simulink library "dlbsBlockSqrt"  (R2025b)
settings: Solver=VariableStepAuto  StartTime=0.0  StopTime=10.0  RelTol=1e-3
libraries: dlbsBlockExtractGradientGF x1, dlbsBlockInsertGradientGF x1
settings Model: Creator=lt6037  LastModifiedBy=lt6037

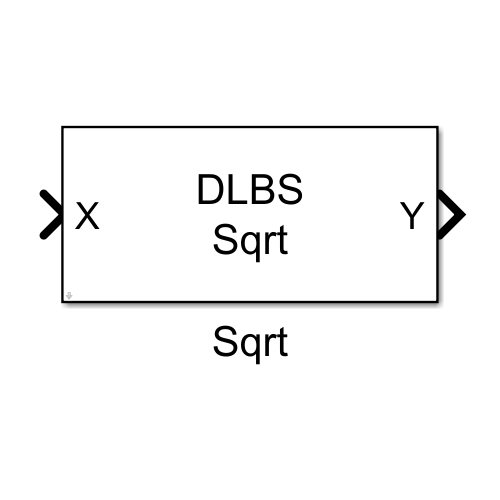
[thumbnail: Simulink's stored preview of the top-level diagram]
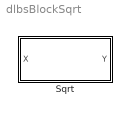
== system dlbsBlockSqrt ==
  Sqrt : Subsystem
      mask help: Applies the square root to the input tensor. The operation is applied element-wise across all tensor elements.
      mask Help: web("dlbsHelpBlockSqrt.html")
      mask Display: fprintf("DLBS\nSqrt");

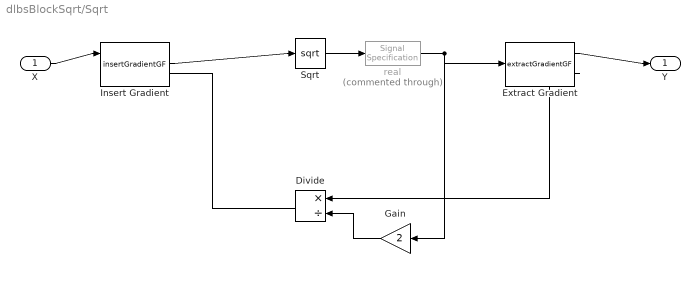
== system dlbsBlockSqrt/Sqrt ==
  X : Inport
  Divide : Product  Inputs=*/
  Extract Gradient : dlbsBlockExtractGradientGF/extractGradientGF
  Gain : Gain  Gain=2
  Insert Gradient : dlbsBlockInsertGradientGF/insertGradientGF
  Sqrt : Sqrt
  real : SignalSpecification  Commented=through
  Y : Outport
  wires:
  Insert Gradient/1 -> Sqrt/1
  Sqrt/1 -> real/1
  Divide/1 -> Insert Gradient/2
  Extract Gradient/2 -> Divide/1
  Gain/1 -> Divide/2
  real/1 -> Extract Gradient/1, Gain/1
  Extract Gradient/1 -> Y/1
  X/1 -> Insert Gradient/1
